simulink model "Sim_Modell_RFJ"  (R2020b)
settings: Solver=VariableStepAuto  StartTime=0.0  StopTime=10.0  RelTol=1e-3
undefined symbols (not defined in the file or in its folder): ACD120_80_Rotor, ACD120_80_Stator, Ausleger, Auslegerplatte, DistanzhuelseGP, Federbolzen, Grundplatte, Heidenhain_ERN_1080, Lagerdeckel_oben, Lagerdeckel_unten, par_imp, par_reg, parSys, Seitenplatte, Visualisierung, Welle, X, Y, Z
libraries: sm_lib x37, fl_lib x7, nesl_utility x7, cstblocks x2, simulink x1
(part 3 of 3)

== matlab function Sim_Modell_RFJ/Subsystem/Backstepping ==
  data: xx input; ML input; u output; par_soll input; act input; parSys parameter; par_reg parameter; ML_est output
function [u,ML_est]= Backstepping(xx, ML, par_soll, act, parSys, par_reg)

    Ia = parSys.I_a;
    da = parSys.d_a;
    c0 = parSys.c_0;
    
    k1 = par_reg.k1;
    gamma = par_reg.gamma1;
    
    d = par_soll(1);
    M_max = par_soll(2);
    c = par_soll(3);
    
    x11 = xx(1);
    x12 = xx(2);
    x2 = xx(3);
    
    % Mometnt berechnen
    M = M_max*tanh(c*x11/M_max);
    dM = c * (0.1e1 - tanh(c * x11 / M_max) ^ 2);
    
    
    % Maple import
    g2 = 1;
    f2 = 0;
    dalpha = [-1 / c0 * dM + 1 -1 / c0 * (d - da);];
    x1p = [x12 0.1e1 / Ia * (-c0 * x11 - da * x12 + ML) + 0.1e1 / Ia * c0 * x2];
    dV1 = [M - ML Ia * x12;];
    gg1 = [0 0.1e1 / Ia * c0];
    alpha = -0.1e1 / c0 * (M + x12 * (d - da)) + x11;


    u = 1/g2*(-f2 + dalpha*x1p' - 1/gamma * dV1*gg1' - k1*(x2-alpha));
    ML_est = ML;

== matlab function Sim_Modell_RFJ/system (nonlinear)/MATLAB Function ==
  data: x input; omegat input; ML input; xp output
function xp = fcn(x, omegat, ML)
    xp = zeros(3,1);
    xp = RFJ_Student(x, omegat, ML);
end

== matlab function Sim_Modell_RFJ/system (nonlinear)/MATLAB Function1 ==
  data: x input; y output; parSys parameter
function y = fcn(x, parSys)

y = zeros(3,1); % necesary for home

% map the states
phit=x(1);
phia=x(2);
omega=x(3);

% create the output
y(1) = phia;
y(2) = omega;
y(3) = phit;

== matlab function Sim_Modell_RFJ/Subsystem/Backstepping_Adaptiv ==
  settings: updateMethod=DISCRETE  sampleTime=0.001
  data: xx input; u output; par_soll input; act input; parSys parameter; par_reg parameter; ML_est output
function [u,ML_est]= Backstepping(xx, par_soll, act, parSys, par_reg)

persistent ML_dach
if isempty(ML_dach) ML_dach = 0; end

Ia = parSys.I_a;
da = parSys.d_a;
c0 = parSys.c_0;

k0 = par_reg.k0;
k1 = par_reg.k1;
gamma = par_reg.gamma1;
Ta = par_reg.Ta;

d = par_soll(1);
M_max = par_soll(2);
c = par_soll(3);

x11 = xx(1);
x12 = xx(2);
x2 = xx(3);

% Moment berechnen
M = M_max*tanh(c*x11/M_max);
dM = c * (0.1e1 - tanh(c * x11 / M_max) ^ 2);

% Maple import
g2 = 1;
f2 = 0;
dalpha = [-1 / c0 * dM + 1 -1 / c0 * (d - da);];
x1p = [x12 0.1e1 / Ia * (-c0 * x11 - da * x12 + ML_dach) + 0.1e1 / Ia * c0 * x2];
dV1 = [M - ML_dach Ia * x12;];
gg1 = [0 0.1e1 / Ia * c0];
alpha = -0.1e1 / c0 * (M + x12 * (d - da)) + x11;

% Stellgesetz
if act
    u = 1/g2*(-f2 + dalpha*x1p' - 1/gamma * dV1*gg1' - k1*(x2-alpha));
else
    u = 0;
end

% Schätzer
if act
    dML = [0, 1/Ia] * k0/gamma*(dV1'-gamma*(x2-alpha)*dalpha');
    ML_dach = ML_dach + dML*Ta;
    ML_est = ML_dach;
else
    ML_dach = 0;
    ML_est = 0;
end
